simulink model "simulacion"  (R2015b)
settings: Solver=VariableStepAuto  StartTime=0.0  StopTime=60*60*3  RelTol=1e-3
values from neighbouring files (symbols this model uses):
  A = [[-(h_12 * A_12 + h_15 * A_15),          h_12 * A_12          ,               0              ,      0      , h_15 * A_15] ./ (c_1 * m_1), ... (first row only)    [p1.m]
  B = transp([1, 0, 0, 0, 0])    [p1.m]
  C = [[1, 0, 0, 0, 0], ... (first row only)    [p1.m]
  U = alpha * Phi    (= 5)    [p1.m]
  x_0 = transp([294.15, 291.15, 294.15, 285.15, 294.15])    [p1.m]
settings Model: Creator=mytorojas  LastModifiedBy=mytorojas

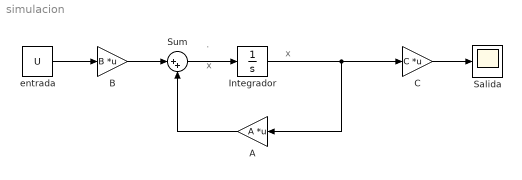
== system simulacion ==
  note: .
  note: x
  note: x
  A : Gain  Gain=A  Multiplication=Matrix(K*u)
  B : Gain  Gain=B  Multiplication=Matrix(K*u)
  C : Gain  Gain=C  Multiplication=Matrix(K*u)
  Integrador : Integrator  InitialCondition=x_0
  Salida : Scope
  Sum : Sum  Inputs=|++
  entrada : Constant  Value=U
  wires:
  entrada/1 -> B/1
  Integrador/1 -> C/1, A/1
  A/1 -> Sum/2
  B/1 -> Sum/1
  Sum/1 -> Integrador/1
  C/1 -> Salida/1
